simulink model "test_shading_control"  (R2016b)
settings: Solver=ode45  StartTime=180*24*3600  StopTime=190*24*3600  RelTol=1e-3  EnableMultiTasking=on
undefined symbols (not defined in the file): path_carnot
libraries: carnot x3, simulink x1
settings Model: Creator=drhf  LastModifiedBy=drhf
settings DataIOCC: LimitDataPoints=on  SaveFormat=Array  SignalLoggingSaveFormat=ModelDataLogs
settings OptimizationCC: ExpressionDepthLimit=2147483647  LifeSpan=inf
settings DebuggingCC: UnderspecifiedInitializationDetection=Classic  MergeDetectMultiDrivingBlocksExec=none  SolverPrmCheckMsg=warning  StateNameClashWarn=warning  SFUnexpectedBacktrackingDiag=warning  SFNoUnconditionalDefaultTransitionDiag=warning  SFExecutionAtInitializationDiag=none
settings HardwareCC: ProdBitPerPointer=32  ProdBitPerSizeT=32  ProdBitPerPtrDiffT=32  ProdLargestAtomicFloat=None  ProdIntDivRoundTo=Undefined  ProdEndianess=Unspecified  ProdWordSize=32  ProdHWDeviceType=32-bit Generic
settings ModelReferenceCC: PropagateSignalLabelsOutOfModel=off
settings GRTTargetCC: TargetLangStandard=C89/C90 (ANSI)  GeneratePreprocessorConditionals=Disable all  CombineOutputUpdateFcns=off  GRTInterface=on
settings ConfigComp: CovMetricSettings=dw  CovHtmlReporting=on  CovSaveCumulativeToWorkspaceVar=on  CovSaveSingleToWorkspaceVar=on  CovExternalEMLEnable=off

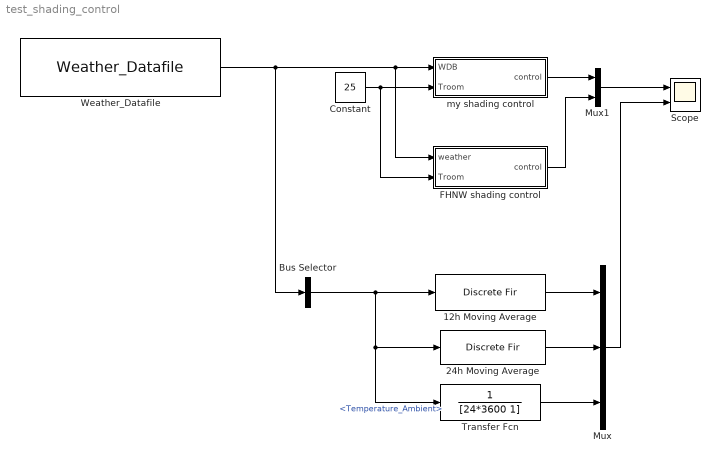
== system test_shading_control ==
  12h Moving Average : DiscreteFir  Coefficients=ones(1,12)*(1/12)  SampleTime=3600  AccumDataTypeStr=Inherit: Same as product output  RndMeth=Nearest
  24h Moving Average : DiscreteFir  Coefficients=ones(1,24)*(1/24)  SampleTime=3600  AccumDataTypeStr=Inherit: Same as product output  RndMeth=Nearest
  Bus Selector : BusSelector  OutputSignals=Temperature_Ambient
  Constant : Constant  Value=25
  FHNW shading control : Subsystem
  Mux : Mux  Inputs=3
  Mux1 : Mux  Inputs=2
  Scope : Scope  NumInputPorts=2
  Transfer Fcn : TransferFcn  Denominator=[24*3600 1]
  Weather_Datafile : carnot/Weather/Weather_Datafile  PathName=path_carnot('data')  FileName='DE_TRY2010_12_averageYear.mat'  UserParam=off  VariableName=DE_TRY2010_12_averageYear  SampleTime=3600
  my shading control : Subsystem
  wires:
  Bus Selector/1 -> 12h Moving Average/1, Transfer Fcn/1, 24h Moving Average/1  "<Temperature_Ambient>"
  Weather_Datafile/1 -> Bus Selector/1, my shading control/1(WDB), FHNW shading control/1(weather)
  Constant/1 -> my shading control/2(Troom), FHNW shading control/2(Troom)
  12h Moving Average/1 -> Mux/1
  Transfer Fcn/1 -> Mux/3
  Mux/1 -> Scope/2
  my shading control/1(control) -> Mux1/1
  FHNW shading control/1(control) -> Mux1/2
  Mux1/1 -> Scope/1
  24h Moving Average/1 -> Mux/2

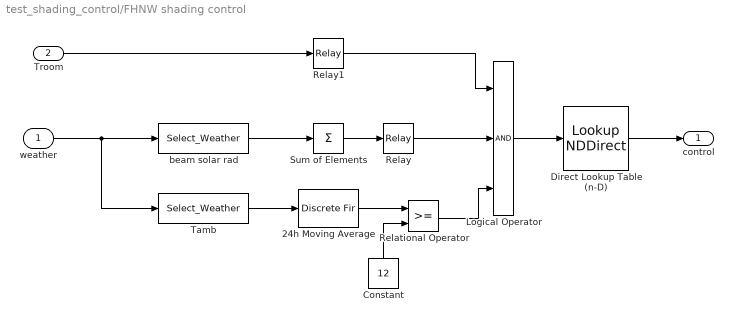
== system test_shading_control/FHNW shading control ==
  weather : Inport
  Troom : Inport  Port=2
  24h Moving Average : DiscreteFir  Coefficients=ones(1,24)*(1/24)  SampleTime=60  AccumDataTypeStr=Inherit: Same as product output  RndMeth=Nearest
  Constant : Constant  Value=12
  Direct Lookup Table (n-D) : LookupNDDirect  NumberOfTableDimensions=1  Table=[1 1-0.75]
  Logical Operator : Logic  Inputs=3  AllPortsSameDT=off  OutDataTypeStr=boolean
  Relational Operator : RelationalOperator  OutDataTypeStr=boolean  RndMeth=Nearest
  Relay : Relay  OnSwitchValue=300  OffSwitchValue=200
  Relay1 : Relay  OnSwitchValue=23.8  OffSwitchValue=22.8
  Sum of Elements : Sum  Inputs=+
  Tamb : carnot/Weather/Select_Weather  v=6
  beam solar rad : carnot/Weather/Select_Weather  v=[17 18]
  control : Outport
  wires:
  beam solar rad/1 -> Sum of Elements/1
  24h Moving Average/1 -> Relational Operator/1
  Logical Operator/1 -> Direct Lookup Table (n-D)/1
  Sum of Elements/1 -> Relay/1
  Relay/1 -> Logical Operator/2
  Relational Operator/1 -> Logical Operator/3
  Troom/1 -> Relay1/1
  Direct Lookup Table (n-D)/1 -> control/1
  weather/1 -> Tamb/1, beam solar rad/1
  Relay1/1 -> Logical Operator/1
  Constant/1 -> Relational Operator/2
  Tamb/1 -> 24h Moving Average/1

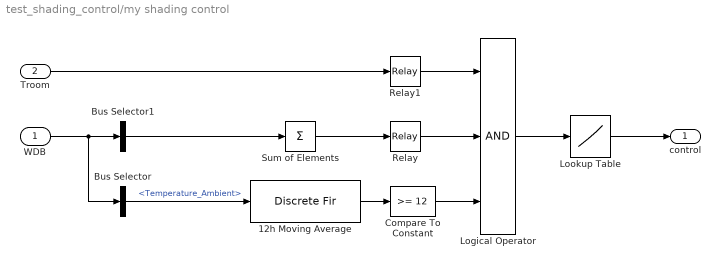
== system test_shading_control/my shading control ==
  WDB : Inport
  Troom : Inport  Port=2
  12h Moving Average : DiscreteFir  Coefficients=ones(1,24)*(1/24)  SampleTime=1800  AccumDataTypeStr=Inherit: Same as product output  RndMeth=Nearest
  Bus Selector : BusSelector  OutputSignals=Temperature_Ambient
  Bus Selector1 : BusSelector  OutputSignals=Solar_Radiation_direct_surface,Solar_Radiation_diffuse_surface  OutputAsBus=on
  Compare To Constant : simulink/Logic and Bit Operations/Compare To Constant  relop=>=  const=12  OutDataTypeStr=uint8
  Logical Operator : Logic  Inputs=3  AllPortsSameDT=off  OutDataTypeStr=boolean
  Lookup Table : Lookup  InputValues=[0 1]  Table=[1 1-0.75]  OutDataTypeStr=double
  Relay : Relay  OnSwitchValue=300  OffSwitchValue=200  OutDataTypeStr=uint8
  Relay1 : Relay  OnSwitchValue=23.8  OffSwitchValue=22.8  OutDataTypeStr=uint8
  Sum of Elements : Sum  Inputs=+
  control : Outport
  wires:
  Bus Selector1/1 -> Sum of Elements/1
  12h Moving Average/1 -> Compare To Constant/1
  Logical Operator/1 -> Lookup Table/1
  Sum of Elements/1 -> Relay/1
  Relay/1 -> Logical Operator/2
  Compare To Constant/1 -> Logical Operator/3
  Troom/1 -> Relay1/1
  Lookup Table/1 -> control/1
  WDB/1 -> Bus Selector1/1, Bus Selector/1
  Relay1/1 -> Logical Operator/1
  Bus Selector/1 -> 12h Moving Average/1  "<Temperature_Ambient>"
